simulink model "DiagramaBloquesLC"  (R2017b)
settings: Solver=VariableStepAuto  StartTime=0.0  StopTime=10.0  RelTol=1e-3
values from neighbouring files (symbols this model uses):
  amplitud = x(3)    [LabControl.m]
  kd = x(7)    [LabControl.m]
  ki = x(6)    [LabControl.m]
  kn = x(8)    [LabControl.m]
  kp = x(5)    [LabControl.m]
  perturbacion = x(4)    [LabControl.m]
  practica = x(1)    [LabControl.m]
  senal = x(2)    [LabControl.m]
undefined symbols (not defined in the file or in its folder): sigbuilder_block
libraries: instrumentlib x2, simulink x1
settings Model: Creator=Administrador  LastModifiedBy=Administrador

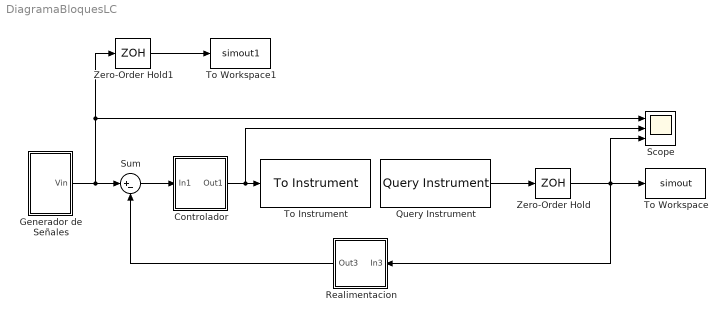
== system DiagramaBloquesLC ==
  Controlador : Subsystem  Tag=PID1  Description=PID
      settings: ErrorFcn=PID
  Generador de Señales : Subsystem
  Query Instrument : instrumentlib/Query Instrument  sampleTime=0.1  isWorkspaceObject=off  timeout=10  inputBufferSize=256  protocol=Serial  serialPort=COM1  baudRate=9600  gpibVendor=Agilent Technologies  boardIndex=0  primaryAddress=1  secondaryAddress=0  visaVendor=Agilent  visaSerialPort=0  chassisIndex=0  logicalAddress=0  tcpRemoteHost='127.0.0.1'  tcpRemotePort=4500  udpRemoteHost='127.0.0.1'  udpRemotePort=9090  visaTCPBoardIndex=0  visaTCPRemoteHost='127.0.0.1'  usbBoardIndex=0  usbManufID=0  usbModelCode=0  usbSerialNumber=0  initAction=None  initCommand='DATA:SOURCE CH1'  initFunction=get  queryCommand='curve?'  responseFormat=ASCII  asciiFormatting='%f'  precision=8-bit integer  byteOrder=Little endian  valuesToRead=1  removeBytes=off  afterOutputAction=Repeat query for new data  enableFrames=off  frameSize=1
      settings: SourceProductName=Instrument Control Toolbox  SourceProductBaseCode=IC
  Realimentacion : Subsystem
  Scope : Scope  NumInputPorts=3
  Sum : Sum  Inputs=|+-
  To Instrument : instrumentlib/To Instrument  sampleTime=0.1  isWorkspaceObject=off  timeout=10  inputBufferSize=256  protocol=Serial  serialPort=COM1  baudRate=9600  gpibVendor=Agilent Technologies  boardIndex=0  primaryAddress=1  secondaryAddress=0  visaVendor=Agilent  visaSerialPort=0  chassisIndex=0  logicalAddress=0  tcpRemoteHost='127.0.0.1'  tcpRemotePort=4500  udpRemoteHost='127.0.0.1'  udpRemotePort=9090  visaTCPBoardIndex=0  visaTCPRemoteHost='127.0.0.1'  usbBoardIndex=0  usbManufID=0  usbModelCode=0  usbSerialNumber=0  initAction=None  initCommand='DATA:SOURCE CH1'  initFunction=get  command=''  sendFormat=ASCII  asciiFormatting='%f'  precision=8-bit integer  byteOrder=Little endian
      settings: SourceProductName=Instrument Control Toolbox  SourceProductBaseCode=IC
  To Workspace : ToWorkspace  VariableName=simout  SaveFormat=Timeseries  SampleTime=-1
  To Workspace1 : ToWorkspace  VariableName=simout1  SaveFormat=Timeseries  SampleTime=-1
  Zero-Order Hold : ZeroOrderHold  SampleTime=0.1
  Zero-Order Hold1 : ZeroOrderHold  SampleTime=0.1
  wires:
  Query Instrument/1 -> Zero-Order Hold/1
  Sum/1 -> Controlador/1("In1 ")
  Controlador/1(Out1) -> Scope/2, To Instrument/1
  Generador de Señales/1("Vin ") -> Zero-Order Hold1/1, Scope/1, Sum/1
  Realimentacion/1(Out3) -> Sum/2
  Zero-Order Hold/1 -> Scope/3, To Workspace/1, Realimentacion/1(In3)
  Zero-Order Hold1/1 -> To Workspace1/1

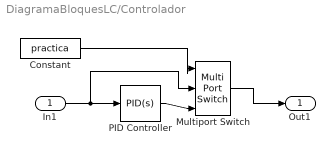
== system DiagramaBloquesLC/Controlador ==
  "In1 " : Inport
  Constant : Constant  Value=practica
  Multiport Switch : MultiPortSwitch  Inputs=2
  PID Controller : simulink/Continuous/PID Controller  Controller=PID  TimeDomain=Continuous-time  SampleTime=-1  IntegratorMethod=Forward Euler  FilterMethod=Forward Euler  Form=Parallel  UseFilter=on  ControllerParametersSource=internal  P=kp  I=ki  D=kd  N=kn  InitialConditionSource=internal  InitialConditionForIntegrator=0  InitialConditionForFilter=0  ExternalReset=none  LimitOutput=off  UpperSaturationLimit=inf  LowerSaturationLimit=-inf  LinearizeAsGain=on  AntiWindupMode=none  Kb=1  TrackingMode=off  Kt=1  PParamMin=[]  PParamMax=[]  IParamMin=[]  IParamMax=[]  DParamMin=[]  DParamMax=[]  NParamMin=[]  NParamMax=[]  KbParamMin=[]  KbParamMax=[]  KtParamMin=[]  KtParamMax=[]  POutMin=[]  POutMax=[]  IOutMin=[]  IOutMax=[]  DOutMin=[]  DOutMax=[]  NOutMin=[]  NOutMax=[]  KbOutMin=[]  KbOutMax=[]  KtOutMin=[]  KtOutMax=[]  IntegratorOutMin=[]  IntegratorOutMax=[]  FilterOutMin=[]  FilterOutMax=[]  SumOutMin=[]  SumOutMax=[]  SumI1OutMin=[]  SumI1OutMax=[]  SumI2OutMin=[]  SumI2OutMax=[]  SumI3OutMin=[]  SumI3OutMax=[]  SumDOutMin=[]  SumDOutMax=[]  SaturationOutMin=[]  SaturationOutMax=[]  IntegratorContinuousStateAttributes=''  IntegratorStateMustResolveToSignalObject=off  IntegratorRTWStateStorageClass=Auto  FilterContinuousStateAttributes=''  FilterStateMustResolveToSignalObject=off  FilterRTWStateStorageClass=Auto  DifferentiatorICPrevScaledInput=0  DifferentiatorOutMin=[]  DifferentiatorOutMax=[]  InitialConditionSetting=State (most efficient)  FilterDiffOutCoefMin=[]  FilterDiffOutCoefMax=[]  SumDenOutMin=[]  SumDenOutMax=[]  SumNumOutMin=[]  SumNumOutMax=[]  ReciprocalOutMin=[]  ReciprocalOutMax=[]  DivideOutMin=[]  DivideOutMax=[]  TunerSelectOption=Transfer Function Based (PID Tuner App)
  Out1 : Outport
  wires:
  "In1 "/1 -> Multiport Switch/2, PID Controller/1
  Constant/1 -> Multiport Switch/1
  Multiport Switch/1 -> Out1/1
  PID Controller/1 -> Multiport Switch/3

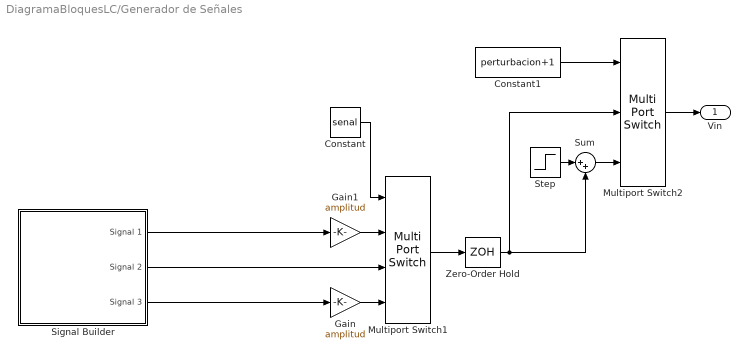
== system DiagramaBloquesLC/Generador de Señales ==
  Constant : Constant  Value=senal
  Constant1 : Constant  Value=perturbacion+1
  Gain : Gain  Gain=amplitud
  Gain1 : Gain  Gain=amplitud
  Multiport Switch1 : MultiPortSwitch
  Multiport Switch2 : MultiPortSwitch  Inputs=2
  Signal Builder : Subsystem  Tag=STV Subsys  LoadFcn=sigbuilder_block('load');  StartFcn=sigbuilder_block('start');  StopFcn=sigbuilder_block('stop');  ClipboardFcn=sigbuilder_block('clipboard');  mask(Sigbuilder block){tuvar=[0:10]}
      mask help: Simulink:masks:SigbuilderBlock_MD
      mask init:
      | if ~strcmp(get_param(bdroot(gcbh),'SimulationStatus'),'stopped') tuvar = sigbuilder_block('maskInit'); end
      settings: CopyFcn=sigbuilder_block('copy');  DeleteFcn=sigbuilder_block('delete');  ModelCloseFcn=sigbuilder_block('modelClose');  PreSaveFcn=sigbuilder_block('preSave');  PauseFcn=sigbuilder_block('pause');  ContinueFcn=sigbuilder_block('continue');  NameChangeFcn=sigbuilder_block('namechange');  OpenFcn=sigbuilder_block('open',[6 30 948 639.75 ]);  CloseFcn=sigbuilder_block('close');
      mask Display: plot(0, 0, 100, 100,[2, 2, 32, 32, 2], [68, 8, 8, 68, 68],[32, 2], [38, 38], [32, 19, 2],[53, 60, 44], [32, 17, 17, 2],[16, 16, 31, 31]);txt = getActiveGroup(gcbh);text(2, 100, txt,'verticalAlignment', 'top');
  Step : Step  Time=3  SampleTime=0.1
  Sum : Sum  Inputs=|++
  Zero-Order Hold : ZeroOrderHold  SampleTime=0.1
  "Vin " : Outport
  wires:
  Signal Builder/3(Signal 3) -> Gain/1
  Signal Builder/2(Signal 2) -> Multiport Switch1/3
  Multiport Switch1/1 -> Zero-Order Hold/1
  Signal Builder/1(Signal 1) -> Gain1/1
  Constant/1 -> Multiport Switch1/1
  Gain/1 -> Multiport Switch1/4
  Gain1/1 -> Multiport Switch1/2
  Constant1/1 -> Multiport Switch2/1
  Step/1 -> Sum/1
  Zero-Order Hold/1 -> Multiport Switch2/2, Sum/2
  Multiport Switch2/1 -> "Vin "/1
  Sum/1 -> Multiport Switch2/3

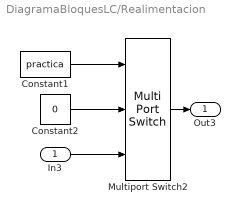
== system DiagramaBloquesLC/Realimentacion ==
  In3 : Inport
  Constant1 : Constant  Value=practica
  Constant2 : Constant  Value=0
  Multiport Switch2 : MultiPortSwitch  Inputs=2
  Out3 : Outport
  wires:
  Constant1/1 -> Multiport Switch2/1
  Multiport Switch2/1 -> Out3/1
  Constant2/1 -> Multiport Switch2/2
  In3/1 -> Multiport Switch2/3

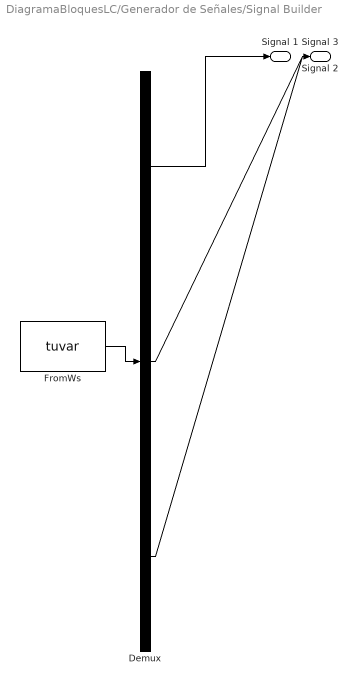
== system DiagramaBloquesLC/Generador de Señales/Signal Builder ==
  Demux : Demux  Tag=STV Demux  Outputs=3
  FromWs : FromWorkspace  Tag=STV FromWs  VariableName=tuvar  SampleTime=0
      SigBuilderData=|
      | common.afterFinalStr = 'Extrapolate'
      | common.sampleTime = 0
      | dataSet.timeRange = [0 10]
      | dataSet.name = 'Group 1'
      | sbobj.Groups.Name = 'Group 1'
      | sbobj.Groups.Signals(1).Name = 'Signal 1'
      | sbobj.Groups.Signals(1).XData = [0 1 1 10]
      | sbobj.Groups.Signals(1).YData = [0 0 1 1]
      | sbobj.Groups.Signals(2).Name = 'Signal 2'
      | sbobj.Groups.Signals(2).XData = [0 1 1 2.98 2.98 4.98 4.98 6.98 6.98 8.98 8.98 10]
      | sbobj.Groups.Signals(2).YData = [0 0 1 1 2 2 3 3 4 4 5 5]
      | sbobj.Groups.Signals(3).Name = 'Signal 3'
      | sbobj.Groups.Signals(3).XData = [0 1 9 10]
      | sbobj.Groups.Signals(3).YData = [0 0 1 1]
  Signal 1 : Outport  Tag=STV Outport
  Signal 2 : Outport  Tag=STV Outport  Port=2
  Signal 3 : Outport  Tag=STV Outport  Port=3
  wires:
  Demux/1 -> Signal 1/1
  FromWs/1 -> Demux/1
  Demux/2 -> Signal 2/1
  Demux/3 -> Signal 3/1
